simulink subsystem "ScanBlock"  (R2025a)
settings: Solver=VariableStepAuto  StartTime=0.0  StopTime=10.0  RelTol=1e-3
model mask{F0=grid.frequency, Theta0=0, Kp_LF=pll.kp, Ki_LF=pll.ki, Ts=5e-5, voltage=Base.KV_base_new, voltagedc=0, mva=0, Amplitude=0, Amplitude1=0, Amplitudedc=0, f=0, T=T, Tdis=5, Tend=10, Hold=Yes}
  mask prompts: F0 "physmod:ee:library:comments:control:eeSinusoidalMeasurement:InitialFrequencyHz_MP"; Theta0 "physmod:ee:library:comments:control:eeSinusoidalMeasurement:InitialPhaseAnglerad_MP"; Kp_LF "physmod:ee:library:comments:control:eeSinusoidalMeasurement:LoopFilterProportionalGain_MP"; Ki_LF "physmod:ee:library:comments:control:eeSinusoidalMeasurement:LoopFilterIntegralGain_MP"; Ts "physmod:ee:library:comments:control:eeSinusoidalMeasurement:SampleTime1ForInherited_MP"; voltage "Base Voltage AC (Volts)"; voltagedc "Base Voltage DC (Volts)"; mva "Base Volt Ampere (VA)"; Amplitude "PRBS Magnitude Along Vd (PU)"; Amplitude1 "PRBS Magnitude Along Vq (PU)"; Amplitudedc "PRBS Magnitude Along Vdc (PU)"; f "Disturbance Frequency Vector (Hz)"; T "Sample Time of PRBS (sec)"; Tdis "Injection Start Time (sec)"; Tend "Injection End Time (sec)"; Hold "Hold Frequency constant During Disturbance"
undefined symbols (not defined in the file): DiscIntNeverNeededParam, ee_sli_rtmsupport, gcbh, w
libraries: slctrl_fre x12, ee_lib x5, eeGeneralControl x4, eeTransforms x4, nesl_utility x3, slctrl_signal x3, simulink x1
(part 2 of 2)

== system ScanBlock/Data Logging for 'frestimate'1/Generate Info Signal/Sinestream ==
  start/stop : Inport
  Info Bus : BusCreator  Inputs=1
  Info Snapshot : slctrl_fre/Frequency Response Estimator/Frequency Response Estimator/Variant Subsystem/PRBSNoEst/Info Snapshot  SystemSampleTime=-1  VariantActivationTime=update diagram  EmptyChoice=off  PassThrough=off  PassThroughVariantControl=(default)  EmptyChoiceVariantControl=(default)  AllowFlexibleInterface=on  Latency=0  AutoFrameSizeCalculation=off
  frequencies : Constant  Value=w  SampleTime=Ts
  Info : Outport
  wires:
  Info Snapshot/1 -> Info Bus/1  "frequencies"
  frequencies/1 -> Info Snapshot/1
  start/stop/1 -> Info Snapshot/Enable
  Info Bus/1 -> Info/1  "Info"

== system ScanBlock/Data Logging for 'frestimate'1/Generate Ready Signal/PRBS ==
  Freq Index : Inport
  Perturbation : Inport  Port=2
  Constant : Constant  Value=0  SampleTime=Ts
  Relational Operator : RelationalOperator  Operator=~=  OutDataTypeStr=boolean  RndMeth=Simplest  InputSameDT=off
  Terminator : Terminator
  Ready : Outport
  wires:
  Relational Operator/1 -> Ready/1  "Ready"
  Constant/1 -> Relational Operator/2
  Perturbation/1 -> Relational Operator/1  "Perturbation"
  Freq Index/1 -> Terminator/1

== system ScanBlock/Data Logging for 'frestimate'1/Generate Ready Signal/Sinestream ==
  Freq Index : Inport
  Perturbation : Inport  Port=2
  ExtractReadySignal : Subsystem  mask(Extract Ready Signal){Ts=Ts, Frequencies=w, NumOfSetPeriod=1, NumOfEstPeriod=2}
      mask prompts: Ts "Sample Time (Ts)"; Frequencies "Frequencies Vector"; NumOfSetPeriod "Number of Settling Periods"; NumOfEstPeriod "Number of Estimation Periods"
      mask help: Extract ready signal for the Sinestream Signal Generator block for offline frequency response estimation.
      mask init:
      | nw = length(Frequencies);
  Terminator : Terminator
  Ready : Outport
  wires:
  Freq Index/1 -> ExtractReadySignal/1(Frequency Index)
  Perturbation/1 -> Terminator/1
  ExtractReadySignal/1(Ready Signal) -> Ready/1  "Ready"

== system ScanBlock/Data Logging for 'frestimate'1/Subtract Nominal Values/Enabled Subsystem ==
  u : Inport
  y : Inport  Port=2
  start/stop : Inport  Port=3
  Enable : EnablePort
  ExtractNominalValues : Subsystem  mask(Remove Nominal Signal){Ts=Ts}
      mask prompts: Ts "Samplt Time (sec)"
      mask help: Remove nominal baseline signal from logged data.
  Sum : Sum  Inputs=|+-
  Sum1 : Sum  Inputs=-+|
  PlantInput : Outport
  PlantOutput : Outport  Port=2
  wires:
  Sum1/1 -> PlantOutput/1
  y/1 -> ExtractNominalValues/2(y), Sum1/2
  ExtractNominalValues/2(yNominal) -> Sum1/1
  u/1 -> ExtractNominalValues/1(u), Sum/1
  ExtractNominalValues/1(uNominal) -> Sum/2
  Sum/1 -> PlantInput/1
  start/stop/1 -> ExtractNominalValues/3(start/stop)

== system ScanBlock/Data Logging for 'frestimate'2/Generate Info Signal/PRBS ==
  start/stop : Inport
  Info Bus : BusCreator  Inputs=1
  Info Snapshot : slctrl_fre/Frequency Response Estimator/Frequency Response Estimator/Variant Subsystem/PRBSNoEst/Info Snapshot  SystemSampleTime=-1  VariantActivationTime=update diagram  EmptyChoice=off  PassThrough=off  PassThroughVariantControl=(default)  EmptyChoiceVariantControl=(default)  AllowFlexibleInterface=on  Latency=0  AutoFrameSizeCalculation=off
  PRBSNumPeriods : Constant  SampleTime=Ts
  Info : Outport
  wires:
  PRBSNumPeriods/1 -> Info Snapshot/1
  Info Bus/1 -> Info/1  "Info"
  Info Snapshot/1 -> Info Bus/1  "PRBSNumPeriods"
  start/stop/1 -> Info Snapshot/Enable

== system ScanBlock/Data Logging for 'frestimate'2/Generate Info Signal/Sinestream ==
  start/stop : Inport
  Info Bus : BusCreator  Inputs=1
  Info Snapshot : slctrl_fre/Frequency Response Estimator/Frequency Response Estimator/Variant Subsystem/PRBSNoEst/Info Snapshot  SystemSampleTime=-1  VariantActivationTime=update diagram  EmptyChoice=off  PassThrough=off  PassThroughVariantControl=(default)  EmptyChoiceVariantControl=(default)  AllowFlexibleInterface=on  Latency=0  AutoFrameSizeCalculation=off
  frequencies : Constant  Value=w  SampleTime=Ts
  Info : Outport
  wires:
  Info Snapshot/1 -> Info Bus/1  "frequencies"
  frequencies/1 -> Info Snapshot/1
  start/stop/1 -> Info Snapshot/Enable
  Info Bus/1 -> Info/1  "Info"

== system ScanBlock/Data Logging for 'frestimate'2/Generate Ready Signal/PRBS ==
  Freq Index : Inport
  Perturbation : Inport  Port=2
  Constant : Constant  Value=0  SampleTime=Ts
  Relational Operator : RelationalOperator  Operator=~=  OutDataTypeStr=boolean  RndMeth=Simplest  InputSameDT=off
  Terminator : Terminator
  Ready : Outport
  wires:
  Relational Operator/1 -> Ready/1  "Ready"
  Constant/1 -> Relational Operator/2
  Perturbation/1 -> Relational Operator/1  "Perturbation"
  Freq Index/1 -> Terminator/1

== system ScanBlock/Data Logging for 'frestimate'2/Generate Ready Signal/Sinestream ==
  Freq Index : Inport
  Perturbation : Inport  Port=2
  ExtractReadySignal : Subsystem  mask(Extract Ready Signal){Ts=Ts, Frequencies=w, NumOfSetPeriod=1, NumOfEstPeriod=2}
      mask prompts: Ts "Sample Time (Ts)"; Frequencies "Frequencies Vector"; NumOfSetPeriod "Number of Settling Periods"; NumOfEstPeriod "Number of Estimation Periods"
      mask help: Extract ready signal for the Sinestream Signal Generator block for offline frequency response estimation.
      mask init:
      | nw = length(Frequencies);
  Terminator : Terminator
  Ready : Outport
  wires:
  Freq Index/1 -> ExtractReadySignal/1(Frequency Index)
  Perturbation/1 -> Terminator/1
  ExtractReadySignal/1(Ready Signal) -> Ready/1  "Ready"

== system ScanBlock/Data Logging for 'frestimate'2/Subtract Nominal Values/Enabled Subsystem ==
  u : Inport
  y : Inport  Port=2
  start/stop : Inport  Port=3
  Enable : EnablePort
  ExtractNominalValues : Subsystem  mask(Remove Nominal Signal){Ts=Ts}
      mask prompts: Ts "Samplt Time (sec)"
      mask help: Remove nominal baseline signal from logged data.
  Sum : Sum  Inputs=|+-
  Sum1 : Sum  Inputs=-+|
  PlantInput : Outport
  PlantOutput : Outport  Port=2
  wires:
  Sum1/1 -> PlantOutput/1
  y/1 -> ExtractNominalValues/2(y), Sum1/2
  ExtractNominalValues/2(yNominal) -> Sum1/1
  u/1 -> ExtractNominalValues/1(u), Sum/1
  ExtractNominalValues/1(uNominal) -> Sum/2
  Sum/1 -> PlantInput/1
  start/stop/1 -> ExtractNominalValues/3(start/stop)

== system ScanBlock/Data Logging for 'frestimate'3/Generate Info Signal/PRBS ==
  start/stop : Inport
  Info Bus : BusCreator  Inputs=1
  Info Snapshot : slctrl_fre/Frequency Response Estimator/Frequency Response Estimator/Variant Subsystem/PRBSNoEst/Info Snapshot  SystemSampleTime=-1  VariantActivationTime=update diagram  EmptyChoice=off  PassThrough=off  PassThroughVariantControl=(default)  EmptyChoiceVariantControl=(default)  AllowFlexibleInterface=on  Latency=0  AutoFrameSizeCalculation=off
  PRBSNumPeriods : Constant  SampleTime=Ts
  Info : Outport
  wires:
  PRBSNumPeriods/1 -> Info Snapshot/1
  Info Bus/1 -> Info/1  "Info"
  Info Snapshot/1 -> Info Bus/1  "PRBSNumPeriods"
  start/stop/1 -> Info Snapshot/Enable

== system ScanBlock/Data Logging for 'frestimate'3/Generate Info Signal/Sinestream ==
  start/stop : Inport
  Info Bus : BusCreator  Inputs=1
  Info Snapshot : slctrl_fre/Frequency Response Estimator/Frequency Response Estimator/Variant Subsystem/PRBSNoEst/Info Snapshot  SystemSampleTime=-1  VariantActivationTime=update diagram  EmptyChoice=off  PassThrough=off  PassThroughVariantControl=(default)  EmptyChoiceVariantControl=(default)  AllowFlexibleInterface=on  Latency=0  AutoFrameSizeCalculation=off
  frequencies : Constant  Value=w  SampleTime=Ts
  Info : Outport
  wires:
  Info Snapshot/1 -> Info Bus/1  "frequencies"
  frequencies/1 -> Info Snapshot/1
  start/stop/1 -> Info Snapshot/Enable
  Info Bus/1 -> Info/1  "Info"

== system ScanBlock/Data Logging for 'frestimate'3/Generate Ready Signal/PRBS ==
  Freq Index : Inport
  Perturbation : Inport  Port=2
  Constant : Constant  Value=0  SampleTime=Ts
  Relational Operator : RelationalOperator  Operator=~=  OutDataTypeStr=boolean  RndMeth=Simplest  InputSameDT=off
  Terminator : Terminator
  Ready : Outport
  wires:
  Relational Operator/1 -> Ready/1  "Ready"
  Constant/1 -> Relational Operator/2
  Perturbation/1 -> Relational Operator/1  "Perturbation"
  Freq Index/1 -> Terminator/1

== system ScanBlock/Data Logging for 'frestimate'3/Generate Ready Signal/Sinestream ==
  Freq Index : Inport
  Perturbation : Inport  Port=2
  ExtractReadySignal : Subsystem  mask(Extract Ready Signal){Ts=Ts, Frequencies=w, NumOfSetPeriod=1, NumOfEstPeriod=2}
      mask prompts: Ts "Sample Time (Ts)"; Frequencies "Frequencies Vector"; NumOfSetPeriod "Number of Settling Periods"; NumOfEstPeriod "Number of Estimation Periods"
      mask help: Extract ready signal for the Sinestream Signal Generator block for offline frequency response estimation.
      mask init:
      | nw = length(Frequencies);
  Terminator : Terminator
  Ready : Outport
  wires:
  Freq Index/1 -> ExtractReadySignal/1(Frequency Index)
  Perturbation/1 -> Terminator/1
  ExtractReadySignal/1(Ready Signal) -> Ready/1  "Ready"

== system ScanBlock/Data Logging for 'frestimate'3/Subtract Nominal Values/Enabled Subsystem ==
  u : Inport
  y : Inport  Port=2
  start/stop : Inport  Port=3
  Enable : EnablePort
  ExtractNominalValues : Subsystem  mask(Remove Nominal Signal){Ts=Ts}
      mask prompts: Ts "Samplt Time (sec)"
      mask help: Remove nominal baseline signal from logged data.
  Scope : Scope  NumInputPorts=2
      settings: ActiveDisplayYMinimum=-8.2439  ActiveDisplayYMaximum=-4.7337  DataLoggingVariableName=ScopeData5
  Sum : Sum  Inputs=|+-
  Sum1 : Sum  Inputs=-+|
  PlantInput : Outport
  PlantOutput : Outport  Port=2
  wires:
  Sum1/1 -> PlantOutput/1, Scope/2
  y/1 -> ExtractNominalValues/2(y), Sum1/2, Scope/1
  ExtractNominalValues/2(yNominal) -> Sum1/1
  u/1 -> ExtractNominalValues/1(u), Sum/1
  ExtractNominalValues/1(uNominal) -> Sum/2
  Sum/1 -> PlantInput/1
  start/stop/1 -> ExtractNominalValues/3(start/stop)

== system ScanBlock/Data Logging for 'frestimate'4/Generate Info Signal/PRBS ==
  start/stop : Inport
  Info Bus : BusCreator  Inputs=1
  Info Snapshot : slctrl_fre/Frequency Response Estimator/Frequency Response Estimator/Variant Subsystem/PRBSNoEst/Info Snapshot  SystemSampleTime=-1  VariantActivationTime=update diagram  EmptyChoice=off  PassThrough=off  PassThroughVariantControl=(default)  EmptyChoiceVariantControl=(default)  AllowFlexibleInterface=on  Latency=0  AutoFrameSizeCalculation=off
  PRBSNumPeriods : Constant  SampleTime=Ts
  Info : Outport
  wires:
  PRBSNumPeriods/1 -> Info Snapshot/1
  Info Bus/1 -> Info/1  "Info"
  Info Snapshot/1 -> Info Bus/1  "PRBSNumPeriods"
  start/stop/1 -> Info Snapshot/Enable

== system ScanBlock/Data Logging for 'frestimate'4/Generate Info Signal/Sinestream ==
  start/stop : Inport
  Info Bus : BusCreator  Inputs=1
  Info Snapshot : slctrl_fre/Frequency Response Estimator/Frequency Response Estimator/Variant Subsystem/PRBSNoEst/Info Snapshot  SystemSampleTime=-1  VariantActivationTime=update diagram  EmptyChoice=off  PassThrough=off  PassThroughVariantControl=(default)  EmptyChoiceVariantControl=(default)  AllowFlexibleInterface=on  Latency=0  AutoFrameSizeCalculation=off
  frequencies : Constant  Value=w  SampleTime=Ts
  Info : Outport
  wires:
  Info Snapshot/1 -> Info Bus/1  "frequencies"
  frequencies/1 -> Info Snapshot/1
  start/stop/1 -> Info Snapshot/Enable
  Info Bus/1 -> Info/1  "Info"

== system ScanBlock/Data Logging for 'frestimate'4/Generate Ready Signal/PRBS ==
  Freq Index : Inport
  Perturbation : Inport  Port=2
  Constant : Constant  Value=0  SampleTime=Ts
  Relational Operator : RelationalOperator  Operator=~=  OutDataTypeStr=boolean  RndMeth=Simplest  InputSameDT=off
  Terminator : Terminator
  Ready : Outport
  wires:
  Relational Operator/1 -> Ready/1  "Ready"
  Constant/1 -> Relational Operator/2
  Perturbation/1 -> Relational Operator/1  "Perturbation"
  Freq Index/1 -> Terminator/1

== system ScanBlock/Data Logging for 'frestimate'4/Generate Ready Signal/Sinestream ==
  Freq Index : Inport
  Perturbation : Inport  Port=2
  ExtractReadySignal : Subsystem  mask(Extract Ready Signal){Ts=Ts, Frequencies=w, NumOfSetPeriod=1, NumOfEstPeriod=2}
      mask prompts: Ts "Sample Time (Ts)"; Frequencies "Frequencies Vector"; NumOfSetPeriod "Number of Settling Periods"; NumOfEstPeriod "Number of Estimation Periods"
      mask help: Extract ready signal for the Sinestream Signal Generator block for offline frequency response estimation.
      mask init:
      | nw = length(Frequencies);
  Terminator : Terminator
  Ready : Outport
  wires:
  Freq Index/1 -> ExtractReadySignal/1(Frequency Index)
  Perturbation/1 -> Terminator/1
  ExtractReadySignal/1(Ready Signal) -> Ready/1  "Ready"

== system ScanBlock/Data Logging for 'frestimate'4/Subtract Nominal Values/Enabled Subsystem ==
  u : Inport
  y : Inport  Port=2
  start/stop : Inport  Port=3
  Enable : EnablePort
  ExtractNominalValues : Subsystem  mask(Remove Nominal Signal){Ts=Ts}
      mask prompts: Ts "Samplt Time (sec)"
      mask help: Remove nominal baseline signal from logged data.
  Sum : Sum  Inputs=|+-
  Sum1 : Sum  Inputs=-+|
  PlantInput : Outport
  PlantOutput : Outport  Port=2
  wires:
  Sum1/1 -> PlantOutput/1
  y/1 -> ExtractNominalValues/2(y), Sum1/2
  ExtractNominalValues/2(yNominal) -> Sum1/1
  u/1 -> ExtractNominalValues/1(u), Sum/1
  ExtractNominalValues/1(uNominal) -> Sum/2
  Sum/1 -> PlantInput/1
  start/stop/1 -> ExtractNominalValues/3(start/stop)

== system ScanBlock/Data Logging for 'frestimate'5/Generate Info Signal/PRBS ==
  start/stop : Inport
  Info Bus : BusCreator  Inputs=1
  Info Snapshot : slctrl_fre/Frequency Response Estimator/Frequency Response Estimator/Variant Subsystem/PRBSNoEst/Info Snapshot  SystemSampleTime=-1  VariantActivationTime=update diagram  EmptyChoice=off  PassThrough=off  PassThroughVariantControl=(default)  EmptyChoiceVariantControl=(default)  AllowFlexibleInterface=on  Latency=0  AutoFrameSizeCalculation=off
  PRBSNumPeriods : Constant  SampleTime=Ts
  Info : Outport
  wires:
  PRBSNumPeriods/1 -> Info Snapshot/1
  Info Bus/1 -> Info/1  "Info"
  Info Snapshot/1 -> Info Bus/1  "PRBSNumPeriods"
  start/stop/1 -> Info Snapshot/Enable

== system ScanBlock/Data Logging for 'frestimate'5/Generate Info Signal/Sinestream ==
  start/stop : Inport
  Info Bus : BusCreator  Inputs=1
  Info Snapshot : slctrl_fre/Frequency Response Estimator/Frequency Response Estimator/Variant Subsystem/PRBSNoEst/Info Snapshot  SystemSampleTime=-1  VariantActivationTime=update diagram  EmptyChoice=off  PassThrough=off  PassThroughVariantControl=(default)  EmptyChoiceVariantControl=(default)  AllowFlexibleInterface=on  Latency=0  AutoFrameSizeCalculation=off
  frequencies : Constant  Value=w  SampleTime=Ts
  Info : Outport
  wires:
  Info Snapshot/1 -> Info Bus/1  "frequencies"
  frequencies/1 -> Info Snapshot/1
  start/stop/1 -> Info Snapshot/Enable
  Info Bus/1 -> Info/1  "Info"

== system ScanBlock/Data Logging for 'frestimate'5/Generate Ready Signal/PRBS ==
  Freq Index : Inport
  Perturbation : Inport  Port=2
  Constant : Constant  Value=0  SampleTime=Ts
  Relational Operator : RelationalOperator  Operator=~=  OutDataTypeStr=boolean  RndMeth=Simplest  InputSameDT=off
  Terminator : Terminator
  Ready : Outport
  wires:
  Relational Operator/1 -> Ready/1  "Ready"
  Constant/1 -> Relational Operator/2
  Perturbation/1 -> Relational Operator/1  "Perturbation"
  Freq Index/1 -> Terminator/1

== system ScanBlock/Data Logging for 'frestimate'5/Generate Ready Signal/Sinestream ==
  Freq Index : Inport
  Perturbation : Inport  Port=2
  ExtractReadySignal : Subsystem  mask(Extract Ready Signal){Ts=Ts, Frequencies=w, NumOfSetPeriod=1, NumOfEstPeriod=2}
      mask prompts: Ts "Sample Time (Ts)"; Frequencies "Frequencies Vector"; NumOfSetPeriod "Number of Settling Periods"; NumOfEstPeriod "Number of Estimation Periods"
      mask help: Extract ready signal for the Sinestream Signal Generator block for offline frequency response estimation.
      mask init:
      | nw = length(Frequencies);
  Terminator : Terminator
  Ready : Outport
  wires:
  Freq Index/1 -> ExtractReadySignal/1(Frequency Index)
  Perturbation/1 -> Terminator/1
  ExtractReadySignal/1(Ready Signal) -> Ready/1  "Ready"

== system ScanBlock/Data Logging for 'frestimate'5/Subtract Nominal Values/Enabled Subsystem ==
  u : Inport
  y : Inport  Port=2
  start/stop : Inport  Port=3
  Enable : EnablePort
  ExtractNominalValues : Subsystem  mask(Remove Nominal Signal){Ts=Ts}
      mask prompts: Ts "Samplt Time (sec)"
      mask help: Remove nominal baseline signal from logged data.
  Sum : Sum  Inputs=|+-
  Sum1 : Sum  Inputs=-+|
  PlantInput : Outport
  PlantOutput : Outport  Port=2
  wires:
  Sum1/1 -> PlantOutput/1
  y/1 -> ExtractNominalValues/2(y), Sum1/2
  ExtractNominalValues/2(yNominal) -> Sum1/1
  u/1 -> ExtractNominalValues/1(u), Sum/1
  ExtractNominalValues/1(uNominal) -> Sum/2
  Sum/1 -> PlantInput/1
  start/stop/1 -> ExtractNominalValues/3(start/stop)

== system ScanBlock/Data Logging for 'frestimate'6/Generate Info Signal/PRBS ==
  start/stop : Inport
  Info Bus : BusCreator  Inputs=1
  Info Snapshot : slctrl_fre/Frequency Response Estimator/Frequency Response Estimator/Variant Subsystem/PRBSNoEst/Info Snapshot  SystemSampleTime=-1  VariantActivationTime=update diagram  EmptyChoice=off  PassThrough=off  PassThroughVariantControl=(default)  EmptyChoiceVariantControl=(default)  AllowFlexibleInterface=on  Latency=0  AutoFrameSizeCalculation=off
  PRBSNumPeriods : Constant  SampleTime=Ts
  Info : Outport
  wires:
  PRBSNumPeriods/1 -> Info Snapshot/1
  Info Bus/1 -> Info/1  "Info"
  Info Snapshot/1 -> Info Bus/1  "PRBSNumPeriods"
  start/stop/1 -> Info Snapshot/Enable

== system ScanBlock/Data Logging for 'frestimate'6/Generate Info Signal/Sinestream ==
  start/stop : Inport
  Info Bus : BusCreator  Inputs=1
  Info Snapshot : slctrl_fre/Frequency Response Estimator/Frequency Response Estimator/Variant Subsystem/PRBSNoEst/Info Snapshot  SystemSampleTime=-1  VariantActivationTime=update diagram  EmptyChoice=off  PassThrough=off  PassThroughVariantControl=(default)  EmptyChoiceVariantControl=(default)  AllowFlexibleInterface=on  Latency=0  AutoFrameSizeCalculation=off
  frequencies : Constant  Value=w  SampleTime=Ts
  Info : Outport
  wires:
  Info Snapshot/1 -> Info Bus/1  "frequencies"
  frequencies/1 -> Info Snapshot/1
  start/stop/1 -> Info Snapshot/Enable
  Info Bus/1 -> Info/1  "Info"

== system ScanBlock/Data Logging for 'frestimate'6/Generate Ready Signal/PRBS ==
  Freq Index : Inport
  Perturbation : Inport  Port=2
  Constant : Constant  Value=0  SampleTime=Ts
  Relational Operator : RelationalOperator  Operator=~=  OutDataTypeStr=boolean  RndMeth=Simplest  InputSameDT=off
  Terminator : Terminator
  Ready : Outport
  wires:
  Relational Operator/1 -> Ready/1  "Ready"
  Constant/1 -> Relational Operator/2
  Perturbation/1 -> Relational Operator/1  "Perturbation"
  Freq Index/1 -> Terminator/1

== system ScanBlock/Data Logging for 'frestimate'6/Generate Ready Signal/Sinestream ==
  Freq Index : Inport
  Perturbation : Inport  Port=2
  ExtractReadySignal : Subsystem  mask(Extract Ready Signal){Ts=Ts, Frequencies=w, NumOfSetPeriod=1, NumOfEstPeriod=2}
      mask prompts: Ts "Sample Time (Ts)"; Frequencies "Frequencies Vector"; NumOfSetPeriod "Number of Settling Periods"; NumOfEstPeriod "Number of Estimation Periods"
      mask help: Extract ready signal for the Sinestream Signal Generator block for offline frequency response estimation.
      mask init:
      | nw = length(Frequencies);
  Terminator : Terminator
  Ready : Outport
  wires:
  Freq Index/1 -> ExtractReadySignal/1(Frequency Index)
  Perturbation/1 -> Terminator/1
  ExtractReadySignal/1(Ready Signal) -> Ready/1  "Ready"

== system ScanBlock/Data Logging for 'frestimate'6/Subtract Nominal Values/Enabled Subsystem ==
  u : Inport
  y : Inport  Port=2
  start/stop : Inport  Port=3
  Enable : EnablePort
  ExtractNominalValues : Subsystem  mask(Remove Nominal Signal){Ts=Ts}
      mask prompts: Ts "Samplt Time (sec)"
      mask help: Remove nominal baseline signal from logged data.
  Sum : Sum  Inputs=|+-
  Sum1 : Sum  Inputs=-+|
  PlantInput : Outport
  PlantOutput : Outport  Port=2
  wires:
  Sum1/1 -> PlantOutput/1
  y/1 -> ExtractNominalValues/2(y), Sum1/2
  ExtractNominalValues/2(yNominal) -> Sum1/1
  u/1 -> ExtractNominalValues/1(u), Sum/1
  ExtractNominalValues/1(uNominal) -> Sum/2
  Sum/1 -> PlantInput/1
  start/stop/1 -> ExtractNominalValues/3(start/stop)

== system ScanBlock/Data Logging for 'frestimate'1/Generate Ready Signal/Sinestream/ExtractReadySignal ==
  Frequency Index : Inport
  Est Period : Constant  Value=NumOfEstPeriod  OutDataTypeStr=double
  MATLAB Function : MATLAB Function  TreatAsAtomicUnit=on
  Numest Scalar Expansion : Gain  Gain=ones(nw,1)
  Numset Scalar Expansion : Gain  Gain=ones(nw,1)
  Set Period : Constant  Value=NumOfSetPeriod  OutDataTypeStr=double
  Triggered Subsystem : Subsystem  TreatAsAtomicUnit=on
  sample time : Constant  Value=Ts  OutDataTypeStr=double
  w constant : Constant  Value=Frequencies  OutDataTypeStr=double
  Ready Signal : Outport
  wires:
  MATLAB Function/3(tsettling) -> Triggered Subsystem/4(tsettling)
  MATLAB Function/2(tstart) -> Triggered Subsystem/3(tstart)
  Set Period/1 -> Numset Scalar Expansion/1
  Triggered Subsystem/1(Ready) -> Ready Signal/1
  Frequency Index/1 -> Triggered Subsystem/Enable, Triggered Subsystem/1(index)
  Numset Scalar Expansion/1 -> MATLAB Function/4(NumOfSetPeriod)
  Est Period/1 -> Numest Scalar Expansion/1
  MATLAB Function/1(Tf) -> Triggered Subsystem/2(Tf)
  w constant/1 -> MATLAB Function/1(Frequencies)
  Numest Scalar Expansion/1 -> MATLAB Function/3(NumOfEstPeriod)
  sample time/1 -> MATLAB Function/2(Ts)

== system ScanBlock/Data Logging for 'frestimate'1/Subtract Nominal Values/Enabled Subsystem/ExtractNominalValues ==
  u : Inport
  y : Inport  Port=2
  start/stop : Inport  Port=3
  DisplayU0 : Display
  DisplayY0 : Display
  Enabled Delay U : Delay  DelayLength=1  InitialConditionSource=Input port  ExternalReset=Rising  SampleTime=Ts
      settings: InputPortMap=u0,r5,p4
  Enabled Delay Y : Delay  DelayLength=1  InitialConditionSource=Input port  ExternalReset=Rising  SampleTime=Ts
      settings: InputPortMap=u0,r5,p4
  uNominal : Outport  OutDataTypeStr=double  VectorParamsAs1DForOutWhenUnconnected=off
  yNominal : Outport  Port=2  OutDataTypeStr=double  VectorParamsAs1DForOutWhenUnconnected=off
  wires:
  y/1 -> Enabled Delay Y/3
  u/1 -> Enabled Delay U/3
  start/stop/1 -> Enabled Delay U/2, Enabled Delay Y/2
  Enabled Delay Y/1 -> DisplayY0/1, Enabled Delay Y/1, yNominal/1  "y"
  Enabled Delay U/1 -> Enabled Delay U/1, DisplayU0/1, uNominal/1  "u"

== system ScanBlock/Data Logging for 'frestimate'2/Generate Ready Signal/Sinestream/ExtractReadySignal ==
  Frequency Index : Inport
  Est Period : Constant  Value=NumOfEstPeriod  OutDataTypeStr=double
  MATLAB Function : MATLAB Function  TreatAsAtomicUnit=on
  Numest Scalar Expansion : Gain  Gain=ones(nw,1)
  Numset Scalar Expansion : Gain  Gain=ones(nw,1)
  Set Period : Constant  Value=NumOfSetPeriod  OutDataTypeStr=double
  Triggered Subsystem : Subsystem  TreatAsAtomicUnit=on
  sample time : Constant  Value=Ts  OutDataTypeStr=double
  w constant : Constant  Value=Frequencies  OutDataTypeStr=double
  Ready Signal : Outport
  wires:
  MATLAB Function/3(tsettling) -> Triggered Subsystem/4(tsettling)
  MATLAB Function/2(tstart) -> Triggered Subsystem/3(tstart)
  Set Period/1 -> Numset Scalar Expansion/1
  Triggered Subsystem/1(Ready) -> Ready Signal/1
  Frequency Index/1 -> Triggered Subsystem/Enable, Triggered Subsystem/1(index)
  Numset Scalar Expansion/1 -> MATLAB Function/4(NumOfSetPeriod)
  Est Period/1 -> Numest Scalar Expansion/1
  MATLAB Function/1(Tf) -> Triggered Subsystem/2(Tf)
  w constant/1 -> MATLAB Function/1(Frequencies)
  Numest Scalar Expansion/1 -> MATLAB Function/3(NumOfEstPeriod)
  sample time/1 -> MATLAB Function/2(Ts)

== system ScanBlock/Data Logging for 'frestimate'2/Subtract Nominal Values/Enabled Subsystem/ExtractNominalValues ==
  u : Inport
  y : Inport  Port=2
  start/stop : Inport  Port=3
  DisplayU0 : Display
  DisplayY0 : Display
  Enabled Delay U : Delay  DelayLength=1  InitialConditionSource=Input port  ExternalReset=Rising  SampleTime=Ts
      settings: InputPortMap=u0,r5,p4
  Enabled Delay Y : Delay  DelayLength=1  InitialConditionSource=Input port  ExternalReset=Rising  SampleTime=Ts
      settings: InputPortMap=u0,r5,p4
  uNominal : Outport  OutDataTypeStr=double  VectorParamsAs1DForOutWhenUnconnected=off
  yNominal : Outport  Port=2  OutDataTypeStr=double  VectorParamsAs1DForOutWhenUnconnected=off
  wires:
  y/1 -> Enabled Delay Y/3
  u/1 -> Enabled Delay U/3
  start/stop/1 -> Enabled Delay U/2, Enabled Delay Y/2
  Enabled Delay Y/1 -> DisplayY0/1, Enabled Delay Y/1, yNominal/1  "y"
  Enabled Delay U/1 -> Enabled Delay U/1, DisplayU0/1, uNominal/1  "u"

== system ScanBlock/Data Logging for 'frestimate'3/Generate Ready Signal/Sinestream/ExtractReadySignal ==
  Frequency Index : Inport
  Est Period : Constant  Value=NumOfEstPeriod  OutDataTypeStr=double
  MATLAB Function : MATLAB Function  TreatAsAtomicUnit=on
  Numest Scalar Expansion : Gain  Gain=ones(nw,1)
  Numset Scalar Expansion : Gain  Gain=ones(nw,1)
  Set Period : Constant  Value=NumOfSetPeriod  OutDataTypeStr=double
  Triggered Subsystem : Subsystem  TreatAsAtomicUnit=on
  sample time : Constant  Value=Ts  OutDataTypeStr=double
  w constant : Constant  Value=Frequencies  OutDataTypeStr=double
  Ready Signal : Outport
  wires:
  MATLAB Function/3(tsettling) -> Triggered Subsystem/4(tsettling)
  MATLAB Function/2(tstart) -> Triggered Subsystem/3(tstart)
  Set Period/1 -> Numset Scalar Expansion/1
  Triggered Subsystem/1(Ready) -> Ready Signal/1
  Frequency Index/1 -> Triggered Subsystem/Enable, Triggered Subsystem/1(index)
  Numset Scalar Expansion/1 -> MATLAB Function/4(NumOfSetPeriod)
  Est Period/1 -> Numest Scalar Expansion/1
  MATLAB Function/1(Tf) -> Triggered Subsystem/2(Tf)
  w constant/1 -> MATLAB Function/1(Frequencies)
  Numest Scalar Expansion/1 -> MATLAB Function/3(NumOfEstPeriod)
  sample time/1 -> MATLAB Function/2(Ts)

== system ScanBlock/Data Logging for 'frestimate'3/Subtract Nominal Values/Enabled Subsystem/ExtractNominalValues ==
  u : Inport
  y : Inport  Port=2
  start/stop : Inport  Port=3
  DisplayU0 : Display
  DisplayY0 : Display
  Enabled Delay U : Delay  DelayLength=1  InitialConditionSource=Input port  ExternalReset=Rising  SampleTime=Ts
      settings: InputPortMap=u0,r5,p4
  Enabled Delay Y : Delay  DelayLength=1  InitialConditionSource=Input port  ExternalReset=Rising  SampleTime=Ts
      settings: InputPortMap=u0,r5,p4
  uNominal : Outport  OutDataTypeStr=double  VectorParamsAs1DForOutWhenUnconnected=off
  yNominal : Outport  Port=2  OutDataTypeStr=double  VectorParamsAs1DForOutWhenUnconnected=off
  wires:
  y/1 -> Enabled Delay Y/3
  u/1 -> Enabled Delay U/3
  start/stop/1 -> Enabled Delay U/2, Enabled Delay Y/2
  Enabled Delay Y/1 -> DisplayY0/1, Enabled Delay Y/1, yNominal/1  "y"
  Enabled Delay U/1 -> Enabled Delay U/1, DisplayU0/1, uNominal/1  "u"

== system ScanBlock/Data Logging for 'frestimate'4/Generate Ready Signal/Sinestream/ExtractReadySignal ==
  Frequency Index : Inport
  Est Period : Constant  Value=NumOfEstPeriod  OutDataTypeStr=double
  MATLAB Function : MATLAB Function  TreatAsAtomicUnit=on
  Numest Scalar Expansion : Gain  Gain=ones(nw,1)
  Numset Scalar Expansion : Gain  Gain=ones(nw,1)
  Set Period : Constant  Value=NumOfSetPeriod  OutDataTypeStr=double
  Triggered Subsystem : Subsystem  TreatAsAtomicUnit=on
  sample time : Constant  Value=Ts  OutDataTypeStr=double
  w constant : Constant  Value=Frequencies  OutDataTypeStr=double
  Ready Signal : Outport
  wires:
  MATLAB Function/3(tsettling) -> Triggered Subsystem/4(tsettling)
  MATLAB Function/2(tstart) -> Triggered Subsystem/3(tstart)
  Set Period/1 -> Numset Scalar Expansion/1
  Triggered Subsystem/1(Ready) -> Ready Signal/1
  Frequency Index/1 -> Triggered Subsystem/Enable, Triggered Subsystem/1(index)
  Numset Scalar Expansion/1 -> MATLAB Function/4(NumOfSetPeriod)
  Est Period/1 -> Numest Scalar Expansion/1
  MATLAB Function/1(Tf) -> Triggered Subsystem/2(Tf)
  w constant/1 -> MATLAB Function/1(Frequencies)
  Numest Scalar Expansion/1 -> MATLAB Function/3(NumOfEstPeriod)
  sample time/1 -> MATLAB Function/2(Ts)

== system ScanBlock/Data Logging for 'frestimate'4/Subtract Nominal Values/Enabled Subsystem/ExtractNominalValues ==
  u : Inport
  y : Inport  Port=2
  start/stop : Inport  Port=3
  DisplayU0 : Display
  DisplayY0 : Display
  Enabled Delay U : Delay  DelayLength=1  InitialConditionSource=Input port  ExternalReset=Rising  SampleTime=Ts
      settings: InputPortMap=u0,r5,p4
  Enabled Delay Y : Delay  DelayLength=1  InitialConditionSource=Input port  ExternalReset=Rising  SampleTime=Ts
      settings: InputPortMap=u0,r5,p4
  uNominal : Outport  OutDataTypeStr=double  VectorParamsAs1DForOutWhenUnconnected=off
  yNominal : Outport  Port=2  OutDataTypeStr=double  VectorParamsAs1DForOutWhenUnconnected=off
  wires:
  y/1 -> Enabled Delay Y/3
  u/1 -> Enabled Delay U/3
  start/stop/1 -> Enabled Delay U/2, Enabled Delay Y/2
  Enabled Delay Y/1 -> DisplayY0/1, Enabled Delay Y/1, yNominal/1  "y"
  Enabled Delay U/1 -> Enabled Delay U/1, DisplayU0/1, uNominal/1  "u"

== system ScanBlock/Data Logging for 'frestimate'5/Generate Ready Signal/Sinestream/ExtractReadySignal ==
  Frequency Index : Inport
  Est Period : Constant  Value=NumOfEstPeriod  OutDataTypeStr=double
  MATLAB Function : MATLAB Function  TreatAsAtomicUnit=on
  Numest Scalar Expansion : Gain  Gain=ones(nw,1)
  Numset Scalar Expansion : Gain  Gain=ones(nw,1)
  Set Period : Constant  Value=NumOfSetPeriod  OutDataTypeStr=double
  Triggered Subsystem : Subsystem  TreatAsAtomicUnit=on
  sample time : Constant  Value=Ts  OutDataTypeStr=double
  w constant : Constant  Value=Frequencies  OutDataTypeStr=double
  Ready Signal : Outport
  wires:
  MATLAB Function/3(tsettling) -> Triggered Subsystem/4(tsettling)
  MATLAB Function/2(tstart) -> Triggered Subsystem/3(tstart)
  Set Period/1 -> Numset Scalar Expansion/1
  Triggered Subsystem/1(Ready) -> Ready Signal/1
  Frequency Index/1 -> Triggered Subsystem/Enable, Triggered Subsystem/1(index)
  Numset Scalar Expansion/1 -> MATLAB Function/4(NumOfSetPeriod)
  Est Period/1 -> Numest Scalar Expansion/1
  MATLAB Function/1(Tf) -> Triggered Subsystem/2(Tf)
  w constant/1 -> MATLAB Function/1(Frequencies)
  Numest Scalar Expansion/1 -> MATLAB Function/3(NumOfEstPeriod)
  sample time/1 -> MATLAB Function/2(Ts)

== system ScanBlock/Data Logging for 'frestimate'5/Subtract Nominal Values/Enabled Subsystem/ExtractNominalValues ==
  u : Inport
  y : Inport  Port=2
  start/stop : Inport  Port=3
  DisplayU0 : Display
  DisplayY0 : Display
  Enabled Delay U : Delay  DelayLength=1  InitialConditionSource=Input port  ExternalReset=Rising  SampleTime=Ts
      settings: InputPortMap=u0,r5,p4
  Enabled Delay Y : Delay  DelayLength=1  InitialConditionSource=Input port  ExternalReset=Rising  SampleTime=Ts
      settings: InputPortMap=u0,r5,p4
  uNominal : Outport  OutDataTypeStr=double  VectorParamsAs1DForOutWhenUnconnected=off
  yNominal : Outport  Port=2  OutDataTypeStr=double  VectorParamsAs1DForOutWhenUnconnected=off
  wires:
  y/1 -> Enabled Delay Y/3
  u/1 -> Enabled Delay U/3
  start/stop/1 -> Enabled Delay U/2, Enabled Delay Y/2
  Enabled Delay Y/1 -> DisplayY0/1, Enabled Delay Y/1, yNominal/1  "y"
  Enabled Delay U/1 -> Enabled Delay U/1, DisplayU0/1, uNominal/1  "u"

== system ScanBlock/Data Logging for 'frestimate'6/Generate Ready Signal/Sinestream/ExtractReadySignal ==
  Frequency Index : Inport
  Est Period : Constant  Value=NumOfEstPeriod  OutDataTypeStr=double
  MATLAB Function : MATLAB Function  TreatAsAtomicUnit=on
  Numest Scalar Expansion : Gain  Gain=ones(nw,1)
  Numset Scalar Expansion : Gain  Gain=ones(nw,1)
  Set Period : Constant  Value=NumOfSetPeriod  OutDataTypeStr=double
  Triggered Subsystem : Subsystem  TreatAsAtomicUnit=on
  sample time : Constant  Value=Ts  OutDataTypeStr=double
  w constant : Constant  Value=Frequencies  OutDataTypeStr=double
  Ready Signal : Outport
  wires:
  MATLAB Function/3(tsettling) -> Triggered Subsystem/4(tsettling)
  MATLAB Function/2(tstart) -> Triggered Subsystem/3(tstart)
  Set Period/1 -> Numset Scalar Expansion/1
  Triggered Subsystem/1(Ready) -> Ready Signal/1
  Frequency Index/1 -> Triggered Subsystem/Enable, Triggered Subsystem/1(index)
  Numset Scalar Expansion/1 -> MATLAB Function/4(NumOfSetPeriod)
  Est Period/1 -> Numest Scalar Expansion/1
  MATLAB Function/1(Tf) -> Triggered Subsystem/2(Tf)
  w constant/1 -> MATLAB Function/1(Frequencies)
  Numest Scalar Expansion/1 -> MATLAB Function/3(NumOfEstPeriod)
  sample time/1 -> MATLAB Function/2(Ts)

== system ScanBlock/Data Logging for 'frestimate'6/Subtract Nominal Values/Enabled Subsystem/ExtractNominalValues ==
  u : Inport
  y : Inport  Port=2
  start/stop : Inport  Port=3
  DisplayU0 : Display
  DisplayY0 : Display
  Enabled Delay U : Delay  DelayLength=1  InitialConditionSource=Input port  ExternalReset=Rising  SampleTime=Ts
      settings: InputPortMap=u0,r5,p4
  Enabled Delay Y : Delay  DelayLength=1  InitialConditionSource=Input port  ExternalReset=Rising  SampleTime=Ts
      settings: InputPortMap=u0,r5,p4
  uNominal : Outport  OutDataTypeStr=double  VectorParamsAs1DForOutWhenUnconnected=off
  yNominal : Outport  Port=2  OutDataTypeStr=double  VectorParamsAs1DForOutWhenUnconnected=off
  wires:
  y/1 -> Enabled Delay Y/3
  u/1 -> Enabled Delay U/3
  start/stop/1 -> Enabled Delay U/2, Enabled Delay Y/2
  Enabled Delay Y/1 -> DisplayY0/1, Enabled Delay Y/1, yNominal/1  "y"
  Enabled Delay U/1 -> Enabled Delay U/1, DisplayU0/1, uNominal/1  "u"

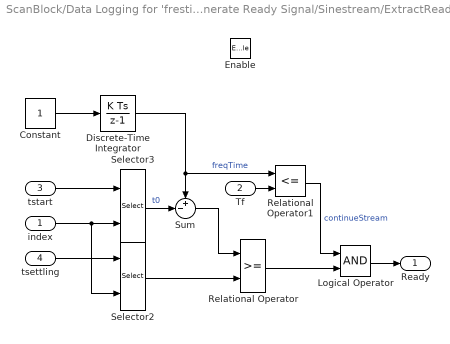
== system ScanBlock/Data Logging for 'frestimate'1/Generate Ready Signal/Sinestream/ExtractReadySignal/Triggered Subsystem ==
  index : Inport
  Tf : Inport  Port=2
  tstart : Inport  Port=3
  tsettling : Inport  Port=4
  Enable : EnablePort
  Constant : Constant  OutDataTypeStr=double
  Discrete-Time Integrator : DiscreteIntegrator  SampleTime=Ts  ICPrevOutput=DiscIntNeverNeededParam  ICPrevScaledInput=DiscIntNeverNeededParam
  Logical Operator : Logic  AllPortsSameDT=off  OutDataTypeStr=boolean
  Relational Operator : RelationalOperator  OutDataTypeStr=boolean  RndMeth=Simplest  InputSameDT=off
  Relational Operator1 : RelationalOperator  Operator=<=  OutDataTypeStr=boolean  RndMeth=Simplest  InputSameDT=off
  Selector2 : Selector  InputPortWidth=nw  IndexOptions=Index vector (port)  Indices=[1 3]  OutputSizes=1
  Selector3 : Selector  InputPortWidth=nw  IndexOptions=Index vector (port)  Indices=[1 3]  OutputSizes=1
  Sum : Sum  Inputs=+-|
  Ready : Outport
  wires:
  Logical Operator/1 -> Ready/1
  Relational Operator1/1 -> Logical Operator/1  "continueStream"
  Tf/1 -> Relational Operator1/2
  Relational Operator/1 -> Logical Operator/2
  index/1 -> Selector3/2, Selector2/2
  Discrete-Time Integrator/1 -> Relational Operator1/1, Sum/1  "freqTime"
  Selector3/1 -> Sum/2  "t0"
  Selector2/1 -> Relational Operator/2
  tsettling/1 -> Selector2/1
  tstart/1 -> Selector3/1
  Sum/1 -> Relational Operator/1
  Constant/1 -> Discrete-Time Integrator/1

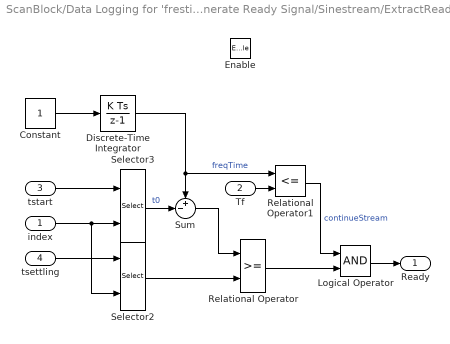
== system ScanBlock/Data Logging for 'frestimate'2/Generate Ready Signal/Sinestream/ExtractReadySignal/Triggered Subsystem ==
  index : Inport
  Tf : Inport  Port=2
  tstart : Inport  Port=3
  tsettling : Inport  Port=4
  Enable : EnablePort
  Constant : Constant  OutDataTypeStr=double
  Discrete-Time Integrator : DiscreteIntegrator  SampleTime=Ts  ICPrevOutput=DiscIntNeverNeededParam  ICPrevScaledInput=DiscIntNeverNeededParam
  Logical Operator : Logic  AllPortsSameDT=off  OutDataTypeStr=boolean
  Relational Operator : RelationalOperator  OutDataTypeStr=boolean  RndMeth=Simplest  InputSameDT=off
  Relational Operator1 : RelationalOperator  Operator=<=  OutDataTypeStr=boolean  RndMeth=Simplest  InputSameDT=off
  Selector2 : Selector  InputPortWidth=nw  IndexOptions=Index vector (port)  Indices=[1 3]  OutputSizes=1
  Selector3 : Selector  InputPortWidth=nw  IndexOptions=Index vector (port)  Indices=[1 3]  OutputSizes=1
  Sum : Sum  Inputs=+-|
  Ready : Outport
  wires:
  Logical Operator/1 -> Ready/1
  Relational Operator1/1 -> Logical Operator/1  "continueStream"
  Tf/1 -> Relational Operator1/2
  Relational Operator/1 -> Logical Operator/2
  index/1 -> Selector3/2, Selector2/2
  Discrete-Time Integrator/1 -> Relational Operator1/1, Sum/1  "freqTime"
  Selector3/1 -> Sum/2  "t0"
  Selector2/1 -> Relational Operator/2
  tsettling/1 -> Selector2/1
  tstart/1 -> Selector3/1
  Sum/1 -> Relational Operator/1
  Constant/1 -> Discrete-Time Integrator/1

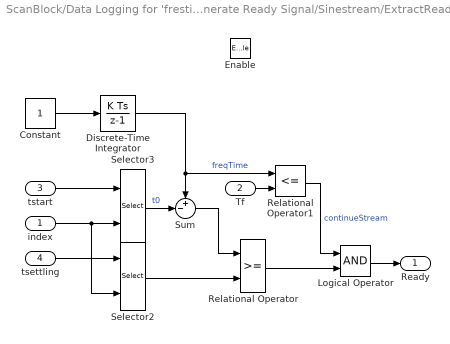
== system ScanBlock/Data Logging for 'frestimate'3/Generate Ready Signal/Sinestream/ExtractReadySignal/Triggered Subsystem ==
  index : Inport
  Tf : Inport  Port=2
  tstart : Inport  Port=3
  tsettling : Inport  Port=4
  Enable : EnablePort
  Constant : Constant  OutDataTypeStr=double
  Discrete-Time Integrator : DiscreteIntegrator  SampleTime=Ts  ICPrevOutput=DiscIntNeverNeededParam  ICPrevScaledInput=DiscIntNeverNeededParam
  Logical Operator : Logic  AllPortsSameDT=off  OutDataTypeStr=boolean
  Relational Operator : RelationalOperator  OutDataTypeStr=boolean  RndMeth=Simplest  InputSameDT=off
  Relational Operator1 : RelationalOperator  Operator=<=  OutDataTypeStr=boolean  RndMeth=Simplest  InputSameDT=off
  Selector2 : Selector  InputPortWidth=nw  IndexOptions=Index vector (port)  Indices=[1 3]  OutputSizes=1
  Selector3 : Selector  InputPortWidth=nw  IndexOptions=Index vector (port)  Indices=[1 3]  OutputSizes=1
  Sum : Sum  Inputs=+-|
  Ready : Outport
  wires:
  Logical Operator/1 -> Ready/1
  Relational Operator1/1 -> Logical Operator/1  "continueStream"
  Tf/1 -> Relational Operator1/2
  Relational Operator/1 -> Logical Operator/2
  index/1 -> Selector3/2, Selector2/2
  Discrete-Time Integrator/1 -> Relational Operator1/1, Sum/1  "freqTime"
  Selector3/1 -> Sum/2  "t0"
  Selector2/1 -> Relational Operator/2
  tsettling/1 -> Selector2/1
  tstart/1 -> Selector3/1
  Sum/1 -> Relational Operator/1
  Constant/1 -> Discrete-Time Integrator/1

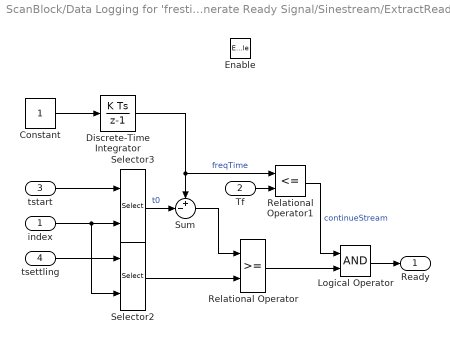
== system ScanBlock/Data Logging for 'frestimate'4/Generate Ready Signal/Sinestream/ExtractReadySignal/Triggered Subsystem ==
  index : Inport
  Tf : Inport  Port=2
  tstart : Inport  Port=3
  tsettling : Inport  Port=4
  Enable : EnablePort
  Constant : Constant  OutDataTypeStr=double
  Discrete-Time Integrator : DiscreteIntegrator  SampleTime=Ts  ICPrevOutput=DiscIntNeverNeededParam  ICPrevScaledInput=DiscIntNeverNeededParam
  Logical Operator : Logic  AllPortsSameDT=off  OutDataTypeStr=boolean
  Relational Operator : RelationalOperator  OutDataTypeStr=boolean  RndMeth=Simplest  InputSameDT=off
  Relational Operator1 : RelationalOperator  Operator=<=  OutDataTypeStr=boolean  RndMeth=Simplest  InputSameDT=off
  Selector2 : Selector  InputPortWidth=nw  IndexOptions=Index vector (port)  Indices=[1 3]  OutputSizes=1
  Selector3 : Selector  InputPortWidth=nw  IndexOptions=Index vector (port)  Indices=[1 3]  OutputSizes=1
  Sum : Sum  Inputs=+-|
  Ready : Outport
  wires:
  Logical Operator/1 -> Ready/1
  Relational Operator1/1 -> Logical Operator/1  "continueStream"
  Tf/1 -> Relational Operator1/2
  Relational Operator/1 -> Logical Operator/2
  index/1 -> Selector3/2, Selector2/2
  Discrete-Time Integrator/1 -> Relational Operator1/1, Sum/1  "freqTime"
  Selector3/1 -> Sum/2  "t0"
  Selector2/1 -> Relational Operator/2
  tsettling/1 -> Selector2/1
  tstart/1 -> Selector3/1
  Sum/1 -> Relational Operator/1
  Constant/1 -> Discrete-Time Integrator/1

== system ScanBlock/Data Logging for 'frestimate'5/Generate Ready Signal/Sinestream/ExtractReadySignal/Triggered Subsystem ==
  index : Inport
  Tf : Inport  Port=2
  tstart : Inport  Port=3
  tsettling : Inport  Port=4
  Enable : EnablePort
  Constant : Constant  OutDataTypeStr=double
  Discrete-Time Integrator : DiscreteIntegrator  SampleTime=Ts  ICPrevOutput=DiscIntNeverNeededParam  ICPrevScaledInput=DiscIntNeverNeededParam
  Logical Operator : Logic  AllPortsSameDT=off  OutDataTypeStr=boolean
  Relational Operator : RelationalOperator  OutDataTypeStr=boolean  RndMeth=Simplest  InputSameDT=off
  Relational Operator1 : RelationalOperator  Operator=<=  OutDataTypeStr=boolean  RndMeth=Simplest  InputSameDT=off
  Selector2 : Selector  InputPortWidth=nw  IndexOptions=Index vector (port)  Indices=[1 3]  OutputSizes=1
  Selector3 : Selector  InputPortWidth=nw  IndexOptions=Index vector (port)  Indices=[1 3]  OutputSizes=1
  Sum : Sum  Inputs=+-|
  Ready : Outport
  wires:
  Logical Operator/1 -> Ready/1
  Relational Operator1/1 -> Logical Operator/1  "continueStream"
  Tf/1 -> Relational Operator1/2
  Relational Operator/1 -> Logical Operator/2
  index/1 -> Selector3/2, Selector2/2
  Discrete-Time Integrator/1 -> Relational Operator1/1, Sum/1  "freqTime"
  Selector3/1 -> Sum/2  "t0"
  Selector2/1 -> Relational Operator/2
  tsettling/1 -> Selector2/1
  tstart/1 -> Selector3/1
  Sum/1 -> Relational Operator/1
  Constant/1 -> Discrete-Time Integrator/1

== system ScanBlock/Data Logging for 'frestimate'6/Generate Ready Signal/Sinestream/ExtractReadySignal/Triggered Subsystem ==
  index : Inport
  Tf : Inport  Port=2
  tstart : Inport  Port=3
  tsettling : Inport  Port=4
  Enable : EnablePort
  Constant : Constant  OutDataTypeStr=double
  Discrete-Time Integrator : DiscreteIntegrator  SampleTime=Ts  ICPrevOutput=DiscIntNeverNeededParam  ICPrevScaledInput=DiscIntNeverNeededParam
  Logical Operator : Logic  AllPortsSameDT=off  OutDataTypeStr=boolean
  Relational Operator : RelationalOperator  OutDataTypeStr=boolean  RndMeth=Simplest  InputSameDT=off
  Relational Operator1 : RelationalOperator  Operator=<=  OutDataTypeStr=boolean  RndMeth=Simplest  InputSameDT=off
  Selector2 : Selector  InputPortWidth=nw  IndexOptions=Index vector (port)  Indices=[1 3]  OutputSizes=1
  Selector3 : Selector  InputPortWidth=nw  IndexOptions=Index vector (port)  Indices=[1 3]  OutputSizes=1
  Sum : Sum  Inputs=+-|
  Ready : Outport
  wires:
  Logical Operator/1 -> Ready/1
  Relational Operator1/1 -> Logical Operator/1  "continueStream"
  Tf/1 -> Relational Operator1/2
  Relational Operator/1 -> Logical Operator/2
  index/1 -> Selector3/2, Selector2/2
  Discrete-Time Integrator/1 -> Relational Operator1/1, Sum/1  "freqTime"
  Selector3/1 -> Sum/2  "t0"
  Selector2/1 -> Relational Operator/2
  tsettling/1 -> Selector2/1
  tstart/1 -> Selector3/1
  Sum/1 -> Relational Operator/1
  Constant/1 -> Discrete-Time Integrator/1

== matlab function ScanBlock/Data Logging for 'frestimate'1/Generate Ready Signal/Sinestream/ExtractReadySignal/MATLAB Function ==
  data: Frequencies input; Tf output; Ts input; NumOfEstPeriod input; NumOfSetPeriod input; tstart output; tsettling output
function [Tf, tstart, tsettling] = extractReadySignal(Frequencies,Ts,NumOfEstPeriod,NumOfSetPeriod)
% obtain the number of periods requested for each frequency
NumPeriods = NumOfEstPeriod + NumOfSetPeriod;
% obtain period time for each frequency
T = 2*pi./Frequencies;
% define experiment length for each frequency (add two samples for CA)
Length = NumPeriods.*T+2*Ts;
% calculate start time stamp for each frequency
CUMSUM = cumsum(Length);
tstart = [0;CUMSUM(1:end-1)];
% calculate the settling duration for each frequency (cannot be zero)
tsettling = [NumOfSetPeriod.*T];
% obtain the stop time for the experiment
Tf = CUMSUM(end);

== matlab function ScanBlock/Data Logging for 'frestimate'2/Generate Ready Signal/Sinestream/ExtractReadySignal/MATLAB Function ==
  data: Frequencies input; Tf output; Ts input; NumOfEstPeriod input; NumOfSetPeriod input; tstart output; tsettling output
function [Tf, tstart, tsettling] = extractReadySignal(Frequencies,Ts,NumOfEstPeriod,NumOfSetPeriod)
% obtain the number of periods requested for each frequency
NumPeriods = NumOfEstPeriod + NumOfSetPeriod;
% obtain period time for each frequency
T = 2*pi./Frequencies;
% define experiment length for each frequency (add two samples for CA)
Length = NumPeriods.*T+2*Ts;
% calculate start time stamp for each frequency
CUMSUM = cumsum(Length);
tstart = [0;CUMSUM(1:end-1)];
% calculate the settling duration for each frequency (cannot be zero)
tsettling = [NumOfSetPeriod.*T];
% obtain the stop time for the experiment
Tf = CUMSUM(end);

== matlab function ScanBlock/Data Logging for 'frestimate'3/Generate Ready Signal/Sinestream/ExtractReadySignal/MATLAB Function ==
  data: Frequencies input; Tf output; Ts input; NumOfEstPeriod input; NumOfSetPeriod input; tstart output; tsettling output
function [Tf, tstart, tsettling] = extractReadySignal(Frequencies,Ts,NumOfEstPeriod,NumOfSetPeriod)
% obtain the number of periods requested for each frequency
NumPeriods = NumOfEstPeriod + NumOfSetPeriod;
% obtain period time for each frequency
T = 2*pi./Frequencies;
% define experiment length for each frequency (add two samples for CA)
Length = NumPeriods.*T+2*Ts;
% calculate start time stamp for each frequency
CUMSUM = cumsum(Length);
tstart = [0;CUMSUM(1:end-1)];
% calculate the settling duration for each frequency (cannot be zero)
tsettling = [NumOfSetPeriod.*T];
% obtain the stop time for the experiment
Tf = CUMSUM(end);

== matlab function ScanBlock/Data Logging for 'frestimate'4/Generate Ready Signal/Sinestream/ExtractReadySignal/MATLAB Function ==
  data: Frequencies input; Tf output; Ts input; NumOfEstPeriod input; NumOfSetPeriod input; tstart output; tsettling output
function [Tf, tstart, tsettling] = extractReadySignal(Frequencies,Ts,NumOfEstPeriod,NumOfSetPeriod)
% obtain the number of periods requested for each frequency
NumPeriods = NumOfEstPeriod + NumOfSetPeriod;
% obtain period time for each frequency
T = 2*pi./Frequencies;
% define experiment length for each frequency (add two samples for CA)
Length = NumPeriods.*T+2*Ts;
% calculate start time stamp for each frequency
CUMSUM = cumsum(Length);
tstart = [0;CUMSUM(1:end-1)];
% calculate the settling duration for each frequency (cannot be zero)
tsettling = [NumOfSetPeriod.*T];
% obtain the stop time for the experiment
Tf = CUMSUM(end);

== matlab function ScanBlock/Data Logging for 'frestimate'5/Generate Ready Signal/Sinestream/ExtractReadySignal/MATLAB Function ==
  data: Frequencies input; Tf output; Ts input; NumOfEstPeriod input; NumOfSetPeriod input; tstart output; tsettling output
function [Tf, tstart, tsettling] = extractReadySignal(Frequencies,Ts,NumOfEstPeriod,NumOfSetPeriod)
% obtain the number of periods requested for each frequency
NumPeriods = NumOfEstPeriod + NumOfSetPeriod;
% obtain period time for each frequency
T = 2*pi./Frequencies;
% define experiment length for each frequency (add two samples for CA)
Length = NumPeriods.*T+2*Ts;
% calculate start time stamp for each frequency
CUMSUM = cumsum(Length);
tstart = [0;CUMSUM(1:end-1)];
% calculate the settling duration for each frequency (cannot be zero)
tsettling = [NumOfSetPeriod.*T];
% obtain the stop time for the experiment
Tf = CUMSUM(end);

== matlab function ScanBlock/Data Logging for 'frestimate'6/Generate Ready Signal/Sinestream/ExtractReadySignal/MATLAB Function ==
  data: Frequencies input; Tf output; Ts input; NumOfEstPeriod input; NumOfSetPeriod input; tstart output; tsettling output
function [Tf, tstart, tsettling] = extractReadySignal(Frequencies,Ts,NumOfEstPeriod,NumOfSetPeriod)
% obtain the number of periods requested for each frequency
NumPeriods = NumOfEstPeriod + NumOfSetPeriod;
% obtain period time for each frequency
T = 2*pi./Frequencies;
% define experiment length for each frequency (add two samples for CA)
Length = NumPeriods.*T+2*Ts;
% calculate start time stamp for each frequency
CUMSUM = cumsum(Length);
tstart = [0;CUMSUM(1:end-1)];
% calculate the settling duration for each frequency (cannot be zero)
tsettling = [NumOfSetPeriod.*T];
% obtain the stop time for the experiment
Tf = CUMSUM(end);
